simulink model "v00_0A_0E"  (R2022b)
settings: Solver=FixedStepDiscrete  StartTime=0.0  StopTime=8000  FixedStep=SampleTime  MaxStep=Contactors_StepTime_msec  RelTol=1e-3  EnableMultiTasking=on
undefined symbols (not defined in the file): A_to_mA, BalancingTempGroup, canChannel, CapacityFactor, CC_Inputs, CellSOC, ChargeState, ContactorsFlags, DiscIntNeverNeededParam, gEN_Contactors_StepTime_msec, Ion, isDynamicCurrentEn, Lithium, maxAllowedImbalance, nCells_parallel, nCells_series, nCellTempGrps, PermanentFailRecoveryTrigger, ProtectionFlags, RBal_ohm, SampleTime, sigbuilder_block, StLineEq_varA, StLineEq_varB, TempSelectForDCL, Thresholds, V_to_mV
libraries: simulink x32, spsIdealSwitchLib x21, spsBatteryLib x20, spsSeriesRLCBranchLib x20, spsVoltageMeasurementLib x20, canmsglib x4, canlib x3, dspstat3 x2, spspowerguiLib x2, spsControlledCurrentSourceLib x1, spsCurrentMeasurementLib x1
(part 1 of 7)
settings Model: SimulationMode=accelerator  PacingRate=447  TunableVars=ntemperaturegroup,nCells_series,nCells_parallel,nCelltemperatureGroups  TunableVarsStorageClass=Auto,Auto,Auto,Auto  TunableVarsTypeQualifier=,,,  Creator=Ujwal's PC  LastModifiedBy=L-638
settings SolverCC: AutoInsertRateTranBlk=on
settings OptimizationCC: DefaultParameterBehavior=Inlined  GainParamInheritBuiltInType=on  UseFloatMulNetSlope=on  DefaultUnderspecifiedDataType=single  InlineInvariantSignals=on  EnhancedBackFolding=on  PassReuseOutputArgsThreshold=0  EfficientFloat2IntCast=on  OptimizeBlockOrder=speed  DifferentSizesBufferReuse=on  OptimizationCustomize=off
settings DebuggingCC: MultiTaskRateTransMsg=warning  IntegerOverflowMsg=error  ParameterOverflowMsg=none  ParameterPrecisionLossMsg=none  ParameterTunabilityLossMsg=error  UnconnectedInputMsg=warning  UnconnectedOutputMsg=warning  UnconnectedLineMsg=warning  BusObjectLabelMismatch=error  SFUnexpectedBacktrackingDiag=warning  SFNoUnconditionalDefaultTransitionDiag=warning  UnderSpecifiedDimensionMsg=warning
settings HardwareCC: ProdBitPerPointer=32  ProdBitPerSizeT=32  ProdBitPerPtrDiffT=32  ProdLargestAtomicInteger=Long  ProdWordSize=32  ProdHWDeviceType=STMicroelectronics->Cortex_M3  TargetLargestAtomicInteger=Long  TargetLargestAtomicFloat=Float  TargetIntDivRoundTo=Zero  TargetEndianess=LittleEndian  TargetHWDeviceType=STMicroelectronics->Cortex_M3  ProdEqTarget=off
settings ModelReferenceCC: EnableRefExpFcnMdlSchedulingChecks=on
settings SFSimCC: MATLABDynamicMemAlloc=off
settings RTWCC: PackageGeneratedCodeAndArtifacts=on  PackageName=ChargingAlgorithm  GenerateReport=on  BuildConfiguration=Faster Runs  LaunchReport=on  CheckMdlBeforeBuild=Warning  DLArmComputeVersion=19.05
settings CodeAppCC: ForceParamTrailComments=on  OperatorAnnotations=on  EnableCustomComments=on
settings GRTTargetCC: MatFileLogging=off
settings ConfigComp: CovScope=ReferencedModels

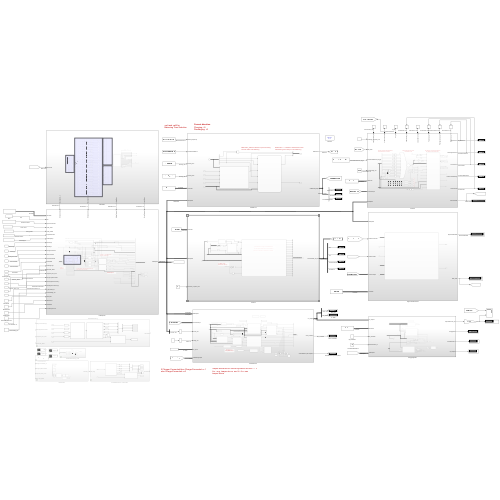
[thumbnail: Simulink's stored preview of the top-level diagram]
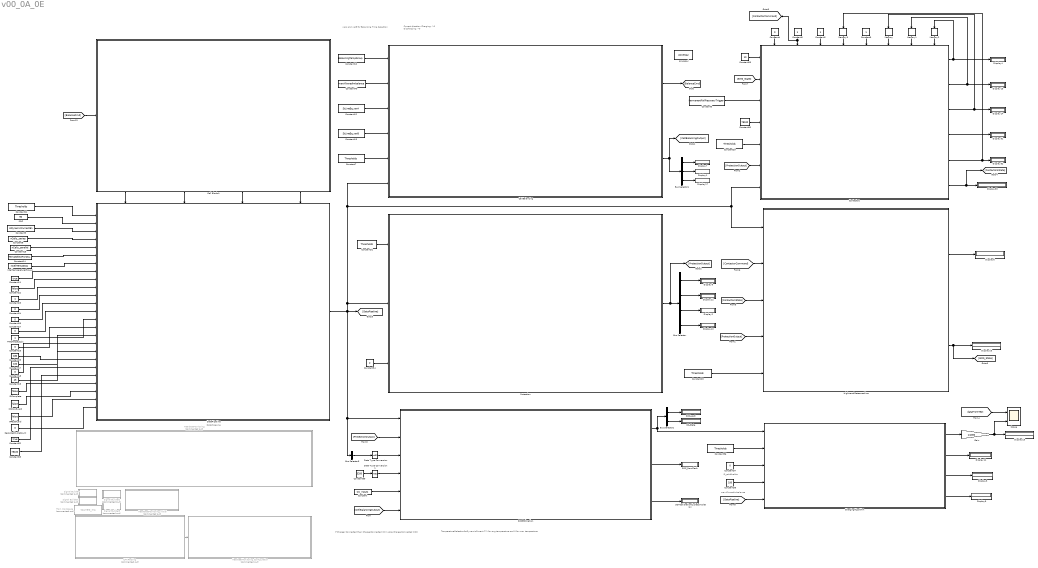
== system v00_0A_0E ==
  note: DataPipeLine
  note: maxAllowedImbalance
  note: IR_calcEnable
  note: Current direction
      | Charging: >0
      | Discharging: <0
  note: TemperatureSelectionforDynamicCurrent = 1 for avg temperature and 0 for max temperature
  note: varA and varB for Balancing Time Selection
  note: If Charger Connected then ChargerConnected == 1 else ChargerConnected ==0
  Bus Selector : BusSelector  OutputSignals=OV,UV,eFuseChargeFlag,ErrorDetect
  Bus Selector1 : BusSelector  OutputSignals=MaxImbalance_mV,BalanceEn,CurrentBalancingState
  Bus Selector2 : BusSelector  OutputSignals=SOC_cpct,CC_State
  Bus Selector3 : BusSelector  OutputSignals=Current_mA
  CAN Packing : Subsystem  Commented=on
  CC_State : Display
  Cell Blocks1 : Subsystem  PartitionName=gEN_Contactors_StepTime_msec  SystemSampleTime=gEN_Contactors_StepTime_msec
      settings: PortSchema="{\"entries\":[{\"content\":{\"sides\":[{\"content\":{\"connectorIds\":[]},\"type\":\"ConnectorPlacement.EquallySpacedRectSide\",\"uuid\":\"5a2a9373-cd4c-4b23-88d3-100c08fcf3ba\"},{\"content\":{\"connectorIds\":[\"In1\"],\"side\":\"RIGHT\"},\"type\":\"ConnectorPlacement.EquallySpacedRectSide\",\"uuid\":\"6030b611-b229-4613-a31e-6d01e62417d7\"},{\"content\":{\"connectorIds\":[],\"side\":\"TOP\"},\"type\":\"ConnectorPlacement.EquallySpacedRectSide\",\"uuid\":\"5428b0ad-0964-4f2b-9e55-734f40119dd9\"},{\"content\":{\"connectorIds\":[\"Out1\",\"Out2\",\"Out3\",\"Out4\"],\"side\":\"BOTTOM\"},\"type\":\"ConnectorPlacement.EquallySpacedRectSide\",\"uuid\":\"9d172f87-e025-48df-9ce8-5c0bb4da28c7\"}]},\"type\":\"ConnectorPlacement.EquallySpacedConnector\",\"uuid\":\"e31cef99-f4d2-4bb8-b841-b685c318bcaf\"}],\"packageUris\":[\"http://schema.mathworks.com/mf0/Connector/R2020b\"],\"version\":\"1.0\"}"
  CellBalancing : Subsystem  PartitionName=gEN_Contactors_StepTime_msec  SystemSampleTime=gEN_Contactors_StepTime_msec
  ChargingAlgorithm : Subsystem
  Constant : Constant  Value=CC_Inputs  OutDataTypeStr=Bus: CC_InputsBus
  Constant10 : Constant  Value=BalancingTempGroup  OutDataTypeStr=int32
  Constant11 : Constant  Value=true  OutDataTypeStr=boolean
  Constant12 : Constant  Value=StLineEq_varA  OutDataTypeStr=int32
  Constant13 : Constant  Value=StLineEq_varB  OutDataTypeStr=int32
  Constant14 : Constant  Value=TempSelectForDCL
  Constant15 : Constant  Value=nCells_parallel  OutDataTypeStr=int8
  Constant{16,18,24,26..27} (5 alike) : Constant  Value=0  OutDataTypeStr=boolean
  Constant17 : Constant  Value=100  OutDataTypeStr=single
  Constant19 : Constant  Value=45  OutDataTypeStr=uint32
  Constant2 : Constant  OutDataTypeStr=uint8
  Constant{7,21,28..29,31,36} (6 alike) : Constant  Value=Thresholds  OutDataTypeStr=Bus: ThresholdsBus
  Constant22 : Constant  Value=false  OutDataTypeStr=boolean
  Constant23 : Constant  OutDataTypeStr=boolean
  Constant25 : Constant  Value=180  OutDataTypeStr=uint32
  Constant3 : Constant  OutDataTypeStr=uint8
  Constant30 : Constant  Value=78100  OutDataTypeStr=int32
  Constant32 : Constant  Value=true  OutDataTypeStr=boolean
  Constant33 : Constant  Value=78100  OutDataTypeStr=int32
  Constant34 : Constant  Value=2
  Constant35 : Constant  Value=10
  Constant37 : Constant  Value=0
  Constant38 : Constant  Value=100
  Constant39 : Constant  Value=3200
  Constant4 : Constant  Value=0  OutDataTypeStr=uint8
  Constant40 : Constant  Value=maxAllowedImbalance
  Constant5 : Constant  OutDataTypeStr=uint8
  Constant6 : Constant  Value=PermanentFailRecoveryTrigger  OutDataTypeStr=boolean
  Constant8 : Constant  Value=nCells_series  OutDataTypeStr=Inherit: Inherit via back propagation
  Constant9 : Constant  Value=isDynamicCurrentEn  OutDataTypeStr=boolean
  Contactors : Subsystem  PartitionName=gEN_Contactors_StepTime_msec  SystemSampleTime=SampleTime
      settings: PortSchema="{\"entries\":[{\"content\":{\"sides\":[{\"content\":{\"connectorIds\":[\"In1\",\"In2\",\"In3\",\"In4\",\"In5\",\"In6\",\"In7\"]},\"type\":\"ConnectorPlacement.EquallySpacedRectSide\",\"uuid\":\"67f6f11a-8aea-432d-9361-9ac63ec44693\"},{\"content\":{\"connectorIds\":[\"Out1\",\"Out2\",\"Out3\",\"Out4\",\"Out5\",\"Out6\"],\"side\":\"RIGHT\"},\"type\":\"ConnectorPlacement.EquallySpacedRectSide\",\"uuid\":\"39853bab-4aa8-482f-878a-e45f7f5446a4\"},{\"content\":{\"connectorIds\":[\"In8\",\"In9\",\"In10\",\"In11\",\"In12\",\"In13\",\"In14\",\"In15\"],\"side\":\"TOP\"},\"type\":\"ConnectorPlacement.EquallySpacedRectSide\",\"uuid\":\"db550e6b-d0a7-4843-a4cf-bd7ca59456b3\"}]},\"type\":\"ConnectorPlacement.EquallySpacedConnector\",\"uuid\":\"abe81cb4-6710-4e45-8e2f-2413695c8381\"}],\"packageUris\":[\"http://schema.mathworks.com/mf0/Connector/R2020b\"],\"version\":\"1.0\"}"
  Data Type Conversion : DataTypeConversion  OutDataTypeStr=int32  SaturateOnIntegerOverflow=off  RndMeth=Floor
  Data Type Conversion1 : DataTypeConversion  OutDataTypeStr=int32  SaturateOnIntegerOverflow=off  RndMeth=Floor
  DataPipeline : Subsystem  PartitionName=gEN_Contactors_StepTime_msec  SystemSampleTime=SampleTime
      settings: PortSchema="{\"entries\":[{\"content\":{\"sides\":[{\"content\":{\"connectorIds\":[\"In1\",\"In2\",\"In3\",\"In4\",\"In5\",\"In6\",\"In7\",\"In8\",\"In9\",\"In10\",\"In11\",\"In12\",\"In13\",\"In14\",\"In15\",\"In16\",\"In17\",\"In18\",\"In19\",\"In20\",\"In21\",\"In22\",\"In23\",\"In24\",\"In25\"]},\"type\":\"ConnectorPlacement.EquallySpacedRectSide\",\"uuid\":\"c1803012-4eae-473f-a7f1-6b2b68065387\"},{\"content\":{\"connectorIds\":[\"Out1\"],\"side\":\"RIGHT\"},\"type\":\"ConnectorPlacement.EquallySpacedRectSide\",\"uuid\":\"31b7d618-748e-421d-b6a8-5a2b53fbaaa3\"},{\"content\":{\"connectorIds\":[\"In26\",\"In27\",\"In28\",\"In29\"],\"side\":\"TOP\"},\"type\":\"ConnectorPlacement.EquallySpacedRectSide\",\"uuid\":\"0f22c0de-6e98-4fa0-8b60-f2fdda6702d2\"}]},\"type\":\"ConnectorPlacement.EquallySpacedConnector\",\"uuid\":\"e1218e22-c24d-4cbf-86f8-150348cec393\"}],\"packageUris\":[\"http://schema.mathworks.com/mf0/Connector/R2020b\"],\"version\":\"1.0\"}"
  Display{1..7,9..17,31..33} (19 alike) : Display
  From Workspace : FromWorkspace  Commented=on  VariableName=tCurrent_mA
  Gain : Gain  Gain=1/1000
  HearbeatMonitoring : Subsystem  Commented=on
      settings: PortSchema="{\"entries\":[{\"content\":{\"sides\":[{\"content\":{\"connectorIds\":[\"In1\"]},\"type\":\"ConnectorPlacement.EquallySpacedRectSide\",\"uuid\":\"c6646334-2ad4-4506-af39-47a9994caedd\"},{\"content\":{\"connectorIds\":[\"In2\",\"In3\",\"In4\",\"In5\"],\"side\":\"RIGHT\"},\"type\":\"ConnectorPlacement.EquallySpacedRectSide\",\"uuid\":\"bd532f8a-cda0-497b-b5de-d9765aeda86f\"},{\"content\":{\"connectorIds\":[],\"side\":\"TOP\"},\"type\":\"ConnectorPlacement.EquallySpacedRectSide\",\"uuid\":\"9d028c67-1d28-4c38-942a-b5f5fcb5898e\"}]},\"type\":\"ConnectorPlacement.EquallySpacedConnector\",\"uuid\":\"11ecd2dc-7bd5-4b21-9cf3-fc90831f4371\"}],\"packageUris\":[\"http://schema.mathworks.com/mf0/Connector/R2020b\"],\"version\":\"1.0\"}"
  HearbeatMonitoring_Configuration : Subsystem  Commented=on
      settings: PortSchema="{\"entries\":[{\"content\":{\"sides\":[{\"content\":{\"connectorIds\":[\"In1\"]},\"type\":\"ConnectorPlacement.EquallySpacedRectSide\",\"uuid\":\"a31c8041-49e1-4625-80d5-5f7afdf5caec\"},{\"content\":{\"connectorIds\":[\"In2\"],\"side\":\"RIGHT\"},\"type\":\"ConnectorPlacement.EquallySpacedRectSide\",\"uuid\":\"0a413807-1fdd-4ffc-9797-e7dca452c824\"},{\"content\":{\"connectorIds\":[],\"side\":\"TOP\"},\"type\":\"ConnectorPlacement.EquallySpacedRectSide\",\"uuid\":\"c3e92d90-cec7-4e35-a91d-3bc3daebcd29\"}]},\"type\":\"ConnectorPlacement.EquallySpacedConnector\",\"uuid\":\"46fea1c4-b9d1-4d1f-98a7-2e36381203df\"}],\"packageUris\":[\"http://schema.mathworks.com/mf0/Connector/R2020b\"],\"version\":\"1.0\"}"
  HeartbeatMonitoring_Initial : Subsystem  Commented=on
  HighLevelStatemachine : Subsystem  PartitionName=gEN_Contactors_StepTime_msec  SystemSampleTime=gEN_Contactors_StepTime_msec
  IRComplete : Constant  Value=false
  IRFastGuard : Constant  Value=false
  IRSlowGuard : Constant  Value=false
  Memory : Memory  InitialCondition=ContactorsFlags.Open  InheritSampleTime=on
  Memory1 : Memory  InitialCondition=ContactorsFlags.Open  InheritSampleTime=on
  Memory2 : Memory  InitialCondition=ContactorsFlags.Open  InheritSampleTime=on
  Memory3 : Memory  InitialCondition=ProtectionFlags.NoError  InheritSampleTime=on
  PreChargeLogic : Constant  OutDataTypeStr=boolean
  Protection : Subsystem  PartitionName=gEN_Contactors_StepTime_msec  SystemSampleTime=gEN_Contactors_StepTime_msec
  RecordedCycleCount : Constant  Value=0  OutDataTypeStr=uint32
  SOC : Constant  Value=90  OutDataTypeStr=int32
  SOCEstimation : Subsystem  PartitionName=gEN_Contactors_StepTime_msec  SystemSampleTime=SampleTime
  SOC_FromFlash : Display
  SOC_cpct : Display
  SOHCalibrationCycleCompletion : Display
  Scope : Scope  NumInputPorts=2
  Signal Builder : Subsystem  Tag=STV Subsys  Commented=on  LoadFcn=sigbuilder_block('load');  StartFcn=sigbuilder_block('start');  StopFcn=sigbuilder_block('stop');  ClipboardFcn=sigbuilder_block('clipboard');  mask(Sigbuilder block){tuvar=[0:10]}
      mask help: Simulink:masks:SigbuilderBlock_MD
      mask init:
      | if ~strcmp(get_param(bdroot(gcbh),'SimulationStatus'),'stopped') tuvar = sigbuilder_block('maskInit'); end
      settings: CopyFcn=sigbuilder_block('copy');  DeleteFcn=sigbuilder_block('delete');  ModelCloseFcn=sigbuilder_block('modelClose');  PreSaveFcn=sigbuilder_block('preSave');  PauseFcn=sigbuilder_block('pause');  ContinueFcn=sigbuilder_block('continue');  NameChangeFcn=sigbuilder_block('namechange');  OpenFcn=sigbuilder_block('open',[198 90.6 550.8 400.2 ]);  CloseFcn=sigbuilder_block('close');
      mask Display: plot(0, 0, 100, 100,[2, 2, 32, 32, 2], [68, 8, 8, 68, 68],[32, 2], [38, 38], [32, 19, 2],[53, 60, 44], [32, 17, 17, 2],[16, 16, 31, 31]);txt = getActiveGroup(gcbh);text(2, 100, txt,'verticalAlignment', 'top');
  Signal Builder1 : Subsystem  Tag=STV Subsys  Commented=on  LoadFcn=sigbuilder_block('load');  StartFcn=sigbuilder_block('start');  StopFcn=sigbuilder_block('stop');  ClipboardFcn=sigbuilder_block('clipboard');  mask(Sigbuilder block){tuvar=[0:10]}
      mask help: Simulink:masks:SigbuilderBlock_MD
      mask init:
      | if ~strcmp(get_param(bdroot(gcbh),'SimulationStatus'),'stopped') tuvar = sigbuilder_block('maskInit'); end
      settings: CopyFcn=sigbuilder_block('copy');  DeleteFcn=sigbuilder_block('delete');  ModelCloseFcn=sigbuilder_block('modelClose');  PreSaveFcn=sigbuilder_block('preSave');  PauseFcn=sigbuilder_block('pause');  ContinueFcn=sigbuilder_block('continue');  NameChangeFcn=sigbuilder_block('namechange');  OpenFcn=sigbuilder_block('open',[374.4 116.4 550.8 400.2 ]);  CloseFcn=sigbuilder_block('close');
      mask Display: plot(0, 0, 100, 100,[2, 2, 32, 32, 2], [68, 8, 8, 68, 68],[32, 2], [38, 38], [32, 19, 2],[53, 60, 44], [32, 17, 17, 2],[16, 16, 31, 31]);txt = getActiveGroup(gcbh);text(2, 100, txt,'verticalAlignment', 'top');
  Signal Builder2 : Subsystem  Tag=STV Subsys  Commented=on  LoadFcn=sigbuilder_block('load');  StartFcn=sigbuilder_block('start');  StopFcn=sigbuilder_block('stop');  ClipboardFcn=sigbuilder_block('clipboard');  mask(Sigbuilder block){tuvar=[0:10]}
      mask help: Simulink:masks:SigbuilderBlock_MD
      mask init:
      | if ~strcmp(get_param(bdroot(gcbh),'SimulationStatus'),'stopped') tuvar = sigbuilder_block('maskInit'); end
      settings: CopyFcn=sigbuilder_block('copy');  DeleteFcn=sigbuilder_block('delete');  ModelCloseFcn=sigbuilder_block('modelClose');  PreSaveFcn=sigbuilder_block('preSave');  PauseFcn=sigbuilder_block('pause');  ContinueFcn=sigbuilder_block('continue');  NameChangeFcn=sigbuilder_block('namechange');  OpenFcn=sigbuilder_block('open',[374.4 116.4 550.8 400.2 ]);  CloseFcn=sigbuilder_block('close');
      mask Display: plot(0, 0, 100, 100,[2, 2, 32, 32, 2], [68, 8, 8, 68, 68],[32, 2], [38, 38], [32, 19, 2],[53, 60, 44], [32, 17, 17, 2],[16, 16, 31, 31]);txt = getActiveGroup(gcbh);text(2, 100, txt,'verticalAlignment', 'top');
  Signal Builder3 : Subsystem  Tag=STV Subsys  Commented=on  LoadFcn=sigbuilder_block('load');  StartFcn=sigbuilder_block('start');  StopFcn=sigbuilder_block('stop');  ClipboardFcn=sigbuilder_block('clipboard');  mask(Sigbuilder block){tuvar=[0:10]}
      mask help: Simulink:masks:SigbuilderBlock_MD
      mask init:
      | if ~strcmp(get_param(bdroot(gcbh),'SimulationStatus'),'stopped') tuvar = sigbuilder_block('maskInit'); end
      settings: CopyFcn=sigbuilder_block('copy');  DeleteFcn=sigbuilder_block('delete');  ModelCloseFcn=sigbuilder_block('modelClose');  PreSaveFcn=sigbuilder_block('preSave');  PauseFcn=sigbuilder_block('pause');  ContinueFcn=sigbuilder_block('continue');  NameChangeFcn=sigbuilder_block('namechange');  OpenFcn=sigbuilder_block('open',[374.4 116.4 550.8 400.2 ]);  CloseFcn=sigbuilder_block('close');
      mask Display: plot(0, 0, 100, 100,[2, 2, 32, 32, 2], [68, 8, 8, 68, 68],[32, 2], [38, 38], [32, 19, 2],[53, 60, 44], [32, 17, 17, 2],[16, 16, 31, 31]);txt = getActiveGroup(gcbh);text(2, 100, txt,'verticalAlignment', 'top');
  nCelltemperatureGroups : Constant  Value=nCellTempGrps
  powergui : spspowerguiLib/powergui  Priority=1  SimulationMode=Discrete  SampleTime=SampleTime  frequency=50  Iterations=50  frequencyindice=0  Pbase=100e6  ErrMax=1e-4  UnitsV=kV  UnitsW=MW  buscounter=0  FunctionMessages=off  echomessages=off  EnableUseOfTLC=off  CurrentSourceSwitches=off  DisableSnubberDevices=off  DisableRonSwitches=off  DisableVfSwitches=off  DisplayEquations=off  AutomaticDiscreteSolvers=off  SolverType=Tustin/Backward Euler (TBE)  Interpol=off  ExternalGateDelay=off  methode=off  Ts=100  x0status=blocks  SPID=on  SwTol=0  HookPort=off  NonlinearTolerance=1e-4  nMaxIteration=100  ContinueOnMaxIteration=off  RestoreLinks=warning  ResistiveCurrentMeasurement=off  Frange=[0:2:500]  Ylog=off  Xlog=on  ShowGrid=off  save=off  variable=ZData  structure=0  ZoomFFT=off  StartTime=0.0  cycles=1  DisplayStyle=1  fundamental=60  FreqAxis=off  MaxFrequency=1000  frequencyindicesteady=1  RmsSteady=1  display=off
  wires:
  SOCEstimation/2(SOC_FromFlash) -> SOC_FromFlash/1  "SOC_FromFlash"
  SOCEstimation/3(SOHCalibrationCycleCompletion) -> SOHCalibrationCycleCompletion/1
  Constant7/1 -> CellBalancing/5(Thresholds)  "Thresholds"
  Data Type Conversion1/1 -> SOCEstimation/4(Voltage_mV)  "Voltage_mV"
  DataPipeline/1(DataPipeline) -> Bus Selector3/1, SOCEstimation/1(DataPipeline), [DataPipeline], HighLevelStatemachine/1(DataPipeline), Contactors/7(DataPipeline), CellBalancing/6(DataPipeline), Protection/2(DataPipeline)  "DataPipeline"
  Constant/1 -> SOCEstimation/5(CC_Inputs)  "CC_Inputs"
  SOCEstimation/1(CC_Outputs) -> ChargingAlgorithm/1(CC_Outputs), Bus Selector2/1  "CC_Outputs"
  Constant22/1 -> DataPipeline/9(FastCharge)  "FastCharge"
  Constant39/1 -> Data Type Conversion1/1
  Bus Selector2/1 -> SOC_cpct/1  "<SOC_cpct>"
  Constant11/1 -> DataPipeline/8(SlowCharge)  "SlowCharge"
  Bus Selector2/2 -> CC_State/1  "<CC_State>"
  Cell Blocks1/4(Temperatures2_C) -> DataPipeline/26(Temperatures2_C)  "Temperatures2_C"
  Constant15/1 -> DataPipeline/5(nCells_Parallel)  "nCells_parallel"
  CellBalancing/2(CellBalancingOutput) -> Bus Selector1/1, [CellBalancingOutput]  "CellBalancingOutput"
  Bus Selector1/3 -> Display17/1  "<CurrentBalancingState>"
  Constant24/1 -> DataPipeline/11(TransmissionFail)  "TransmissionFail"
  Cell Blocks1/2(VoltageSense) -> DataPipeline/28(VoltageSense_mV)  "VoltageSense_mV"
  Constant8/1 -> DataPipeline/4(nCells_Series)  "nCells_series"
  Data Type Conversion/1 -> SOCEstimation/3(Current_mA)
  nCelltemperatureGroups/1 -> DataPipeline/7(nCellTempGrps)  "nCellTempGrps"
  Constant28/1 -> HighLevelStatemachine/5(Thresholds)  "Thresholds"
  Constant14/1 -> DataPipeline/6(TempSelectForDCL)  "TempSelectForDCL"
  Constant12/1 -> CellBalancing/3(StLineEq_varA)  "StLineEq_varA"
  Constant21/1 -> DataPipeline/1(Thresholds)  "Thresholds"
  Constant9/1 -> DataPipeline/3(isDynamicCurrentEn)  "isDynamicCurrentEn"
  Constant13/1 -> CellBalancing/4(StLineEq_varB)  "StLineEq_varB"
  Bus Selector/3 -> Display2/1  "<eFuseChargeFlag>"
  Constant27/1 -> DataPipeline/13(ServiceMode)  "ServiceMode"
  Constant23/1 -> DataPipeline/10(isChargerConnected)  "isChargerConnected"
  HighLevelStatemachine/1(HighLevelStateMode) -> Display6/1  "HighLevelStateMode"
  Bus Selector/2 -> Display12/1  "<UV>"
  Cell Blocks1/1(CurrentSense) -> DataPipeline/29(CurrentSense_mA)  "CurrentSense_mA"
  CellBalancing/1(BalanceCmd) -> [BalanceCmd]  "BalanceCmd"
  Bus Selector/1 -> Display9/1  "<OV>"
  Bus Selector1/2 -> Display1/1  "<BalanceEn>"
  Constant10/1 -> CellBalancing/1(BalancingTempGroup)  "BalancingTempGroup"
  Constant26/1 -> DataPipeline/12(VCUPermanentFail)  "VCUPermanentFail"
  Bus Selector1/1 -> Display7/1  "<MaxImbalance_mV>"
  SOC/1 -> DataPipeline/2(SOC)  "SOC"
  Cell Blocks1/3(Temperatures1_C) -> DataPipeline/27(Temperatures1_C)  "Temperatures1_C"
  [BalanceCmd] -> Cell Blocks1/1(BalanceCmd)  "BalanceCmd"
  Bus Selector3/1 -> Data Type Conversion/1  "<Current_mA>"
  Constant19/1 -> DataPipeline/18(SlowChargersCurrentLimit_A)  "SlowChargersCurrentLimit_A"
  Constant16/1 -> DataPipeline/15(BalanceEn_atRest)  "BalanceEn_atRest"
  Constant18/1 -> DataPipeline/17(EmergencyDisconnectEn)  "EmergencyDisconnectEn"
  Constant17/1 -> DataPipeline/16(LoopTimer_SOC_msec)  "LoopTimer_SOC_msec"
  CAN Packing/1(CAN Msg) -> HearbeatMonitoring_Configuration/2(CAN_Msg)
  Constant25/1 -> DataPipeline/19(FastChargersCurrentLimit_A)  "FastChargersCurrentLimit_A"
  PreChargeLogic/1 -> DataPipeline/14(PreChargeLogic)  "PreChargeLogic"
  Constant30/1 -> Contactors/4(TerminalVoltage_mV)  "TerminalVoltage_mV"
  Constant29/1 -> Contactors/5(Thresholds)  "Thresholds"
  Constant4/1 -> Contactors/8(Communication_Flag)  "Communication_Flag"
  Constant3/1 -> Contactors/9(ContactorCommand), [ContactorCommand]  "ContactorCommand"
  Constant2/1 -> Contactors/10(SC_Flag)  "SC_Flag"
  Memory3/1 -> Contactors/11(PermanentFail_FB)  "PermanentFail_Flag"
  Constant5/1 -> Contactors/12(ContactorError_Flag)  "ContactorError_Flag"
  Memory/1 -> Contactors/13(PosContactors_FB)  "PosContactors_FB"
  Memory1/1 -> Contactors/14(PreChargeContactors_FB)  "PreChargeContactors_FB"
  Memory2/1 -> Contactors/15(NegContactors_FB)  "NegContactors_FB"
  Contactors/5(PermanentFaiil) -> Display32/1, Memory3/1  "PermanentFail"
  Contactors/3(PosContactors) -> Display14/1, Memory/1  "PosContactors"
  Constant6/1 -> Contactors/3(PermanentFailRecoveryTrigger)  "PermanentFailRecoveryTrigger"
  Contactors/4(ContactorsWeldWarning) -> Display31/1  "ContactorsWeldWarning"
  Contactors/2(PreChargeContactors) -> Memory1/1, Display13/1  "PreChargeContactors"
  Contactors/6(ContactorsState) -> Display33/1, [ContactorsState]  "ContactorsState"
  Contactors/1(NegContactors) -> Memory2/1, Display4/1  "NegContactors"
  [CellBalancingOutput] -> SOCEstimation/6(CellBalancingOutput)
  [ProtectionOutput] -> HighLevelStatemachine/4(ProtectionOutput)
  [ProtectionOutput] -> Contactors/6(ProtectionOutput)
  [ProtectionOutput] -> SOCEstimation/2(ProtectionOutput)
  Constant31/1 -> Protection/1(Thresholds)  "Thresholds"
  Bus Selector/4 -> Display10/1  "<ErrorDetect>"
  Constant32/1 -> DataPipeline/20(IR_Calculation_En)  "IR_Calculation_En"
  Constant33/1 -> DataPipeline/21(TerminalVoltage_mV)  "TerminalVoltage_mV"
  [ContactorsState] -> HighLevelStatemachine/3(ContactorsState)
  [ContactorCommand] -> HighLevelStatemachine/2(ContactorCommand)
  Constant34/1 -> Protection/3(Protection_LoopTime_msec)
  Constant35/1 -> Contactors/1(PreCharge_LoopTime_msec)
  HighLevelStatemachine/2(BMS_State) -> [BMS_State], Display16/1
  [BMS_State] -> Contactors/2(BMS_State)
  [DataPipeline] -> ChargingAlgorithm/5(DataPipeline)  "DataPipeline"
  Constant36/1 -> ChargingAlgorithm/2(Thresholds)  "Thresholds"
  ChargingAlgorithm/2(ChargingState) -> Display11/1
  ChargingAlgorithm/1(RequestedCurrent_mA) -> Gain/1
  IRComplete/1 -> DataPipeline/22(IRComplete)
  IRSlowGuard/1 -> DataPipeline/23(IRSlowGuard)
  RecordedCycleCount/1 -> DataPipeline/25(RecordedCycleCount)
  IRFastGuard/1 -> DataPipeline/24(IRFastGuard)
  Gain/1 -> Display15/1, Scope/2
  [dataFromTest] -> Scope/1
  Constant37/1 -> ChargingAlgorithm/3(IR_calcEnable)
  Constant38/1 -> ChargingAlgorithm/4(maxAllowedImb_mv)
  Constant40/1 -> CellBalancing/2(maxAllowedImbalance)
  Protection/1(ProtectionState_Out_bus) -> Bus Selector/1, [ProtectionOutput]  "ProtectionOutput"
  ChargingAlgorithm/3(internalResistance) -> Display3/1
  ChargingAlgorithm/4(IR_Complete) -> Display5/1

== system v00_0A_0E/CAN Packing ==
  ChargersCurrentLimit_A : Inport
  EmergencyDisconnectEn : Inport  Port=2
  LoopTimer_SOC_msec : Inport  Port=3
  BalanceEn_atRest : Inport  Port=4
  CAN Configuration : canlib/CAN Configuration  BlockHandle=17.0004  Device=MathWorks Virtual 1 (Channel 1)  DeviceMenu=MathWorks Virtual 1 (Channel 1)  ObjConstructor=canChannel('MathWorks', 'Virtual 1', 1)  BusSpeed=500000  EnableBitParameters=off  AckMode=Normal
  CAN Pack : canmsglib/CAN Pack  MsgList=(none)  MsgName=CAN Msg  MsgIDType=Standard (11-bit identifier)  MsgIdentifier=5  MsgLength=8  Remote=off  ApplyMinMax=off  BusOutput=on  SignalInfo={ 'ChargersCurrentLimit_A', '0', '8', 'LE', 'unsigned', 'Standard', '0', '1', '0', '-Inf', 'Inf'; 'LoopTimer_SOC_msec', '8', '16', 'LE', 'signed', 'Standard', '0', '1', '0', '-Inf', 'Inf'; 'EmergencyDisconnectEn', '24', '8', 'LE', 'signed', 'Standard', '0', '1', '0', '-Inf', 'Inf'; 'BalanceEn_atRest', '32', '32', 'LE', 'unsigned', 'Standard', '0', '1', '0', '-Inf', 'Inf' }
      settings: LibrarySourceBlock=embeddedtargetslib/Host Communication/CAN Pack  DataFormat=manually specified signals
  CAN Receive : canlib/CAN Receive  BlockHandle=24.0004  Device=MathWorks Virtual 1 (Channel 1)  DeviceMenu=MathWorks Virtual 1 (Channel 1)  ObjConstructor=canChannel('MathWorks', 'Virtual 1', 1)  EnableStandardIDsFilter=off  StdIDsCombo=Allow all  StandardIDs=0  EnableExtendedIDsFilter=off  ExtIDsCombo=Allow all  ExtendedIDs=0  SampleTime=0.1  MsgsPerTimestep=all  InternalFilterUpdateStatus=on  BusOutput=on
  CAN Transmit : canlib/CAN Transmit  BlockHandle=27.0004  Device=MathWorks Virtual 1 (Channel 1)  DeviceMenu=MathWorks Virtual 1 (Channel 1)  ObjConstructor=canChannel('MathWorks', 'Virtual 1', 1)  EnableEventTransmit=off  EnablePeriodicTransmit=on  MessagePeriod=0.100
  Data Type Conversion{2..5} (4 alike) : DataTypeConversion  SaturateOnIntegerOverflow=off  RndMeth=Floor
  Terminator : Terminator
  CAN Msg : Outport
  wires:
  LoopTimer_SOC_msec/1 -> Data Type Conversion4/1
  CAN Pack/1 -> CAN Transmit/1  "CAN Msg"
  Data Type Conversion2/1 -> CAN Pack/1
  CAN Receive/2 -> CAN Msg/1  "CAN Msg"
  Data Type Conversion3/1 -> CAN Pack/3
  Data Type Conversion5/1 -> CAN Pack/4
  CAN Receive/1 -> Terminator/1
  ChargersCurrentLimit_A/1 -> Data Type Conversion2/1
  Data Type Conversion4/1 -> CAN Pack/2
  BalanceEn_atRest/1 -> Data Type Conversion5/1
  EmergencyDisconnectEn/1 -> Data Type Conversion3/1
